simulink model "detector11"  (Simulink 2.20)
settings: Solver=FixedStepDiscrete  StartTime=0.0  StopTime=28800  RelTol=1e-3  AbsTol=1e-6
undefined symbols (not defined in the file): firls
libraries: BufferedDSP x23, WinAudio x1
settings Model: SaveTime=off  SaveOutput=off  ConsistencyChecking=off  RTWPlaceOutputsASAP=off  RTWTemplateMakefile=c:\nfc\matlab\simulink\grt_vc_sgm.tmf  RTWMakeCommand="make_rtw USER_SRCS=\"winmm.lib\" USER_INCLUDES=\"-Ic:\\nfc\\matlab\\Simulink\\BufferedDSP\\src\\rtw\""

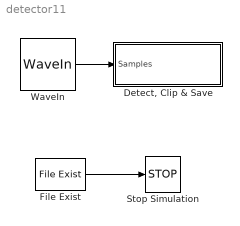
== system detector11 ==
  "Detect, Clip & Save" : Subsystem  mask(DetectClipNSave){buffersize=8192, f0=4000, f1=5500, threshold=2, numChannels=1, col_major=0, fs=22050}
      mask prompts: buffersize "Buffer Size:"; f0 "Lower Frequency (Hz):"; f1 "Upper Frequency (Hz):"; numChannels "Number of Channels:"; col_major "Column major channel order:"; fs "Sample Rate (Hz):"
      mask help: Detects acoustic events in a frequency band, clips, and saves them to disk.
      mask Help: Detects acoustic events in a frequency band, clips, and saves them to disk.
  File Exist : BufferedDSP/Other/File Exist  filename=c:\stop.txt  sampleTime=3*8192/22050
  Stop Simulation : Stop
  WaveIn : WinAudio/WaveIn  sampleRateLit=22050  sampleWidthLit=16  stereo=off  col_major=0  buffersize=8192  bufTime=12
  wires:
  File Exist/1 -> Stop Simulation/1
  WaveIn/1 -> "Detect, Clip & Save"/1(Samples)

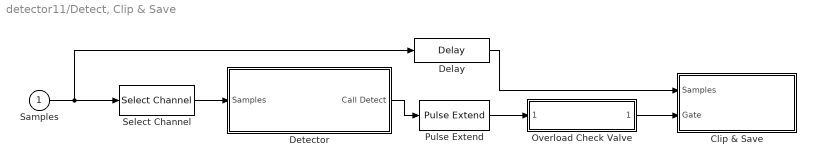
== system detector11/Detect, Clip & Save ==
  Samples : Inport  Port=1  PortWidth=buffersize * numChannels  SampleTime=-1
  Clip & Save : Subsystem  mask(ClipAndSave){buffersize=buffersize, fifosize=buffersize * 4, numChannels=numChannels, col_major=col_major, ftype=Wave, saveDir=c:\temp\calls, fname=Dick, fnamestyle=Time from start, fs=fs}
      mask prompts: buffersize "Buffer size (samples):"; fifosize "FIFO size (samples):"; numChannels "Number of Channels:"; col_major "Column major channel order"; ftype "File type:"; saveDir "Save Directory:"; fname "File Name Prefix:"; fnamestyle "File name time stamp:"; fs "Sample Rate (Hz):"
      mask help: Clips sections from "Samples" according to "Gate" and saves to Save Directory using File Name Prefix and adding a time stamp.
      mask Help: Clips sections from "Samples" according to "Gate" and saves to Save Directory using File Name Prefix and adding a time stamp.
      mask StyleString: edit,edit,edit,edit,popup(Wave|Mac Binary|Matlab|ASCII Float|ASCII Fixed|Binary Float|Binary Fixed|AIFF),edit,edit,popup(GMT|Local time|Time from start),edit
  Delay : BufferedDSP/Memory/Delay  buffersize=buffersize  delay=15000  numChannels=numChannels  col_major=col_major
  Detector : Subsystem  mask(Detector){buffersize=buffersize, f0=f0, f1=f1, filterLength=100, threshold=threshold, numChannels=1, col_major=col_major, fs=fs}
      mask prompts: buffersize "Buffer Size:"; f0 "Lower Frequency (Hz):"; f1 "Upper Frequency (Hz):"; filterLength "Filter Length:"; numChannels "Number of Channels:"; col_major "Column major channel order:"; fs "Sample Rate:"
      mask help: Examines band-limited energy for events.
  Overload Check Valve : Subsystem  mask(Overload Check Valve){buffersize=buffersize, guardTime=20, numEvents=20, fs=fs}
      mask prompts: buffersize "Buffer size (samples):"; guardTime "Length of time to check: (sec)"; numEvents "Prohibited number of events:"; fs "Sample rate (Hz):"
      mask help: Input and output signals are single channel Boolean event markers. If more than a prohibited number of events occur in a specified time duration, the output is zero. Otherwise, the input is passed through (ANDed) to the output.
      mask Help: Input and output signals are single channel Boolean event markers.  If more than a prohibited number of events occur in a specified time duration, the output is zero.  Otherwise, the input is passed through (ANDed) to the output.
      mask Display: disp(sprintf('%d events in %d sec',numEvents,guardTime))
  Pulse Extend : BufferedDSP/Pulse Shapers/Pulse Extend  buffersize=buffersize  lag=10000  numChannels=1  col_major=col_major
  Select Channel : BufferedDSP/Multichannel/Select Channel  buffersize=buffersize  selectChannel=1  numChannels=numChannels  col_major=col_major
  wires:
  Detector/1(Call Detect) -> Pulse Extend/1
  Samples/1 -> Delay/1, Select Channel/1
  Select Channel/1 -> Detector/1(Samples)
  Delay/1 -> Clip & Save/1(Samples)
  Pulse Extend/1 -> Overload Check Valve/1("      ")
  Overload Check Valve/1("     ") -> Clip & Save/2(Gate)

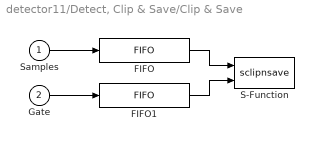
== system detector11/Detect, Clip & Save/Clip & Save ==
  Samples : Inport  Port=1  PortWidth=buffersize * numChannels  SampleTime=-1
  Gate : Inport  Port=2  PortWidth=buffersize  SampleTime=-1
  FIFO : BufferedDSP/Memory/FIFO  input_width=buffersize  output_width=fifosize  numChannels=numChannels  col_major=col_major
  FIFO1 : BufferedDSP/Memory/FIFO  input_width=buffersize  output_width=fifosize  numChannels=1  col_major=col_major
  S-Function : S-Function  FunctionName=sclipnsave  Parameters=buffersize fifosize numChannels col_major fname saveDir ftype fnamestyle fs  PortCounts=[]  SFunctionModules=''
  wires:
  FIFO1/1 -> S-Function/2
  FIFO/1 -> S-Function/1
  Gate/1 -> FIFO1/1
  Samples/1 -> FIFO/1

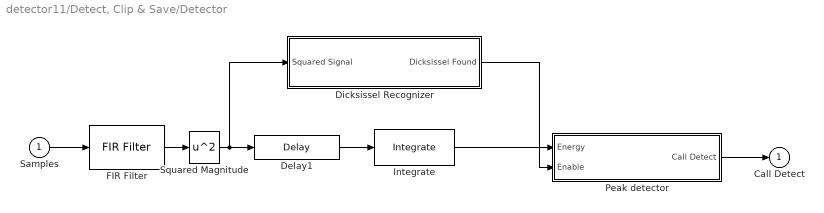
== system detector11/Detect, Clip & Save/Detector ==
  Samples : Inport  Port=1  PortWidth=buffersize *numChannels  SampleTime=-1
  Delay1 : BufferedDSP/Memory/Delay  buffersize=buffersize  delay=10000  numChannels=1  col_major=1
  Dicksissel Recognizer : Subsystem  mask{buffersize=8192, fs=22050, threshold=0.5}
      mask prompts: buffersize "Buffer size:"; fs "Sample Rate (Hz):"
  FIR Filter : BufferedDSP/Filter/Row Major/FIR Filter  input_width=buffersize  nfft_in=2*buffersize  h=firls(filterLength-1,[0 f0-100 f0 f1 f1+100 fs/2]/(fs/2),[0,0,1,1,0,0])  numChannels=numChannels
  Integrate : BufferedDSP/Filter/Integrate  buffersize=buffersize  integration_time=1103  normalize=on  initial_value=0  numChannels=numChannels  col_major=col_major
  Peak detector : Subsystem  mask(PeakDetector){threshold=threshold, buffersize=buffersize, numChannels=numChannels, col_major=col_major, fs=fs}
      mask prompts: buffersize "Buffer Size:"; numChannels "Number of Channels:"; col_major "Column major channel order:"; fs "Sample Rate:"
      mask help: Finds large plateaus in an energy signal.
      mask Help: Finds large plateaus in an energy signal.
  Squared Magnitude : Math  Operator=square
  Call Detect : Outport  Port=1  InitialOutput=0
  wires:
  FIR Filter/1 -> Squared Magnitude/1
  Samples/1 -> FIR Filter/1
  Peak detector/1(Call Detect) -> Call Detect/1
  Squared Magnitude/1 -> Dicksissel Recognizer/1(Squared Signal), Delay1/1
  Dicksissel Recognizer/1(Dicksissel Found) -> Peak detector/2(Enable)
  Delay1/1 -> Integrate/1
  Integrate/1 -> Peak detector/1(Energy)

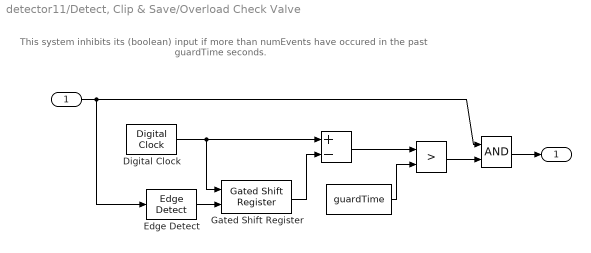
== system detector11/Detect, Clip & Save/Overload Check Valve ==
  note: This system inhibits its (boolean) input if
      | more than numEvents have occured
      | in the past guardTime seconds.
  "      " : Inport  Port=1  PortWidth=buffersize  SampleTime=-1
  " " : Constant  Value=guardTime
  "  " : RelationalOperator  Operator=>
  "    " : Logic  Operator=AND  Inputs=2
  "        " : Sum  Inputs=+-
  Digital Clock : BufferedDSP/Counters/Digital Clock  buffersize=buffersize  t0=guardTime+1  fs=fs
  Edge Detect : BufferedDSP/Pulse Shapers/Edge Detect  buffersize=buffersize  numChannels=1  col_major=1
  Gated Shift Register : BufferedDSP/Memory/Gated Shift Register  buffersize=buffersize  reg_size=numEvents  numChannels=1  col_major=1
  "     " : Outport  Port=1  InitialOutput=0
  wires:
  Digital Clock/1 -> Gated Shift Register/1, "        "/1
  Edge Detect/1 -> Gated Shift Register/2
  Gated Shift Register/1 -> "        "/2
  "        "/1 -> "  "/1
  " "/1 -> "  "/2
  "      "/1 -> "    "/1, Edge Detect/1
  "    "/1 -> "     "/1
  "  "/1 -> "    "/2

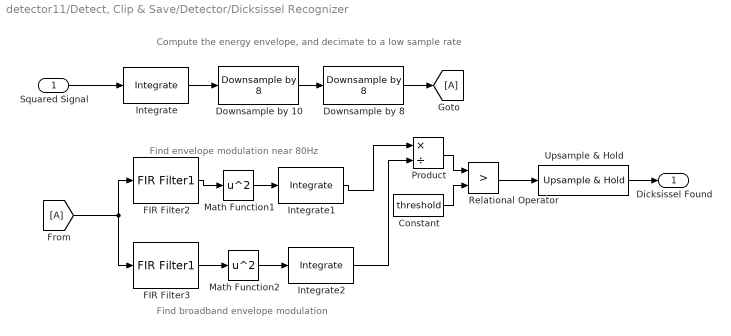
== system detector11/Detect, Clip & Save/Detector/Dicksissel Recognizer ==
  note: Find broadband envelope modulation
  note: Find envelope modulation near 80Hz
  note: Compute the energy envelope, and decimate to a low sample rate
  Squared Signal : Inport  Port=1  PortWidth=buffersize  SampleTime=-1
  Constant : Constant  Value=threshold
  Downsample by 10 : BufferedDSP/Filter/Single Channel/Downsample by 8  buffersize=buffersize  h=fir1(100,1/8)
  Downsample by 8 : BufferedDSP/Filter/Single Channel/Downsample by 8  buffersize=buffersize/8  h=fir1(100,1/8)
  FIR Filter2 : BufferedDSP/Filter/Row Major/FIR Filter1  input_width=buffersize/64  nfft_in=buffersize/32  h=fir1(200,[55,80]/(fs/128),'DC-0')  numChannels=1  Ts=buffersize/fs
  FIR Filter3 : BufferedDSP/Filter/Row Major/FIR Filter1  input_width=buffersize/64  nfft_in=buffersize/32  h=fir1(200,[20,105]/(fs/128),'DC-0')  numChannels=1  Ts=buffersize/fs
  Integrate : BufferedDSP/Filter/Integrate  buffersize=buffersize  integration_time=100  normalize=on  initial_value=0  numChannels=1  col_major=0
  Integrate1 : BufferedDSP/Filter/Integrate  buffersize=buffersize/64  integration_time=round(0.900*fs/64)  normalize=on  initial_value=0  numChannels=1  col_major=0
  Integrate2 : BufferedDSP/Filter/Integrate  buffersize=buffersize/64  integration_time=round(0.900*fs/64)  normalize=on  initial_value=0  numChannels=1  col_major=0
  Math Function1 : Math  Operator=square
  Math Function2 : Math  Operator=square
  Product : Product  Inputs=*/
  Relational Operator : RelationalOperator  Operator=>
  Upsample & Hold : BufferedDSP/Other/Upsample & Hold  buffersize=buffersize/64  L=64
  Dicksissel Found : Outport  Port=1
  wires:
  FIR Filter3/1 -> Math Function2/1
  FIR Filter2/1 -> Math Function1/1
  Downsample by 8/1 -> [A]
  Integrate/1 -> Downsample by 10/1
  Downsample by 10/1 -> Downsample by 8/1
  Squared Signal/1 -> Integrate/1
  Relational Operator/1 -> Upsample & Hold/1
  Upsample & Hold/1 -> Dicksissel Found/1
  Math Function1/1 -> Integrate1/1
  Math Function2/1 -> Integrate2/1
  [A] -> FIR Filter3/1, FIR Filter2/1
  Integrate2/1 -> Product/2
  Integrate1/1 -> Product/1
  Constant/1 -> Relational Operator/2
  Product/1 -> Relational Operator/1

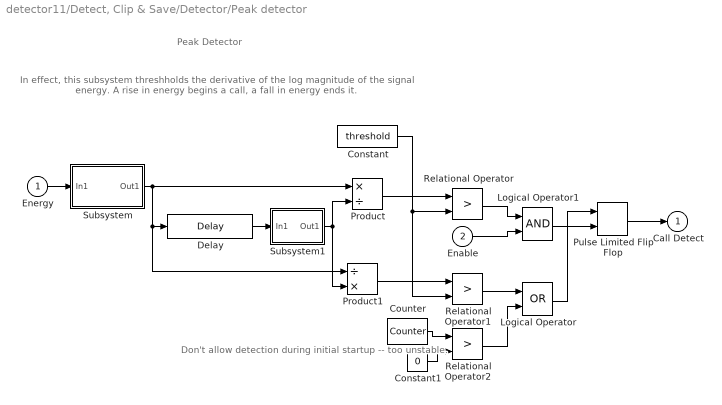
== system detector11/Detect, Clip & Save/Detector/Peak detector ==
  note: Don't allow detection during
      | initial startup -- too unstable.
  note: Peak Detector
  note: In effect, this subsystem threshholds
      | the derivative of the log magnitude
      | of the signal energy.  A rise in energy
      | begins a call, a fall in energy ends it.
  Energy : Inport  Port=1  PortWidth=buffersize * numChannels  SampleTime=-1
  Enable : Inport  Port=2  PortWidth=buffersize  SampleTime=-1
  Constant : Constant  Value=threshold
  Constant1 : Constant  Value=0
  Counter : BufferedDSP/Counters/Counter  buffersize=buffersize  initial_count=1.2*buffersize  count_direction=Down  has_stop_count=on  stop_count=0  numChannels=numChannels  col_major=1  ts=buffersize/fs
  Delay : BufferedDSP/Memory/Delay  buffersize=buffersize  delay=fix(fs * .020)  numChannels=numChannels  col_major=col_major
  Logical Operator : Logic  Operator=OR  Inputs=2
  Logical Operator1 : Logic  Operator=AND  Inputs=2
  Product : Product  Inputs=*/
  Product1 : Product  Inputs=/*
  Pulse Limited Flip Flop : BufferedDSP/Memory/Pulse Limited Flip Flop  buffersize=buffersize  initial_state=0  minLimit=fix(0.1 * fs)  maxLimit=fix(0.4 * fs)  numChannels=numChannels  col_major=col_major
  Relational Operator : RelationalOperator  Operator=>
  Relational Operator1 : RelationalOperator  Operator=>
  Relational Operator2 : RelationalOperator  Operator=>
  Subsystem : Subsystem
      mask Type: Prevent divide-by-zero
      mask Display: disp('Prevent\n divide-by-zero')
  Subsystem1 : Subsystem
      mask Type: Prevent divide-by-zero
      mask Display: disp('Prevent\n divide-by-zero')
  Call Detect : Outport  Port=1  InitialOutput=0
  wires:
  Relational Operator2/1 -> Logical Operator/2
  Constant1/1 -> Relational Operator2/2
  Counter/1 -> Relational Operator2/1
  Relational Operator1/1 -> Logical Operator/1
  Product1/1 -> Relational Operator1/1
  Pulse Limited Flip Flop/1 -> Call Detect/1
  Logical Operator/1 -> Pulse Limited Flip Flop/1
  Relational Operator/1 -> Logical Operator1/1
  Enable/1 -> Logical Operator1/2
  Logical Operator1/1 -> Pulse Limited Flip Flop/2
  Subsystem1/1(Out1) -> Product/2, Product1/2
  Subsystem/1(Out1) -> Product/1, Delay/1, Product1/1
  Delay/1 -> Subsystem1/1(In1)
  Energy/1 -> Subsystem/1(In1)
  Constant/1 -> Relational Operator/2, Relational Operator1/2
  Product/1 -> Relational Operator/1

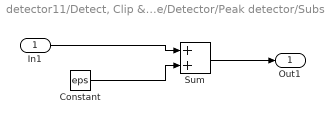
== system detector11/Detect, Clip & Save/Detector/Peak detector/Subsystem ==
  In1 : Inport  Port=1  PortWidth=-1  SampleTime=-1
  Constant : Constant  Value=eps
  Sum : Sum  Inputs=++
  Out1 : Outport  Port=1
  wires:
  Sum/1 -> Out1/1
  Constant/1 -> Sum/2
  In1/1 -> Sum/1

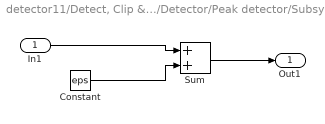
== system detector11/Detect, Clip & Save/Detector/Peak detector/Subsystem1 ==
  In1 : Inport  Port=1  PortWidth=-1  SampleTime=-1
  Constant : Constant  Value=eps
  Sum : Sum  Inputs=++
  Out1 : Outport  Port=1
  wires:
  Sum/1 -> Out1/1
  Constant/1 -> Sum/2
  In1/1 -> Sum/1
